simulink model "clase3"  (R2022b)
settings: Solver=VariableStepAuto  StartTime=0.0  StopTime=10  MaxStep=0.01  RelTol=1e-3
values from neighbouring files (symbols this model uses):
  g = 9.81    [class3.m]
  l1 = 0.3    [class3.m]
  l2 = 0.25    [class3.m]
  m1 = 0.2    [class3.m]
  m2 = 0.1    [class3.m]
settings Model: Creator=nemesis  LastModifiedBy=nemesis

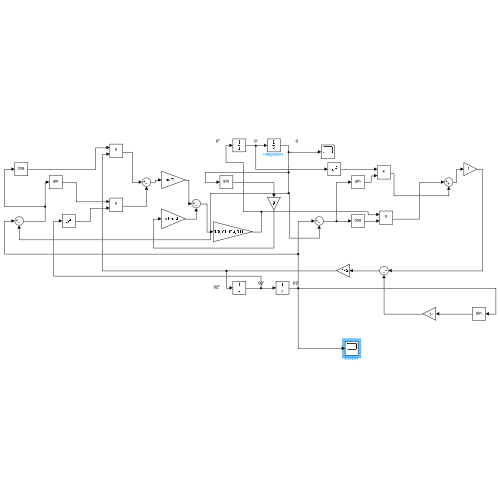
[thumbnail: Simulink's stored preview of the top-level diagram]
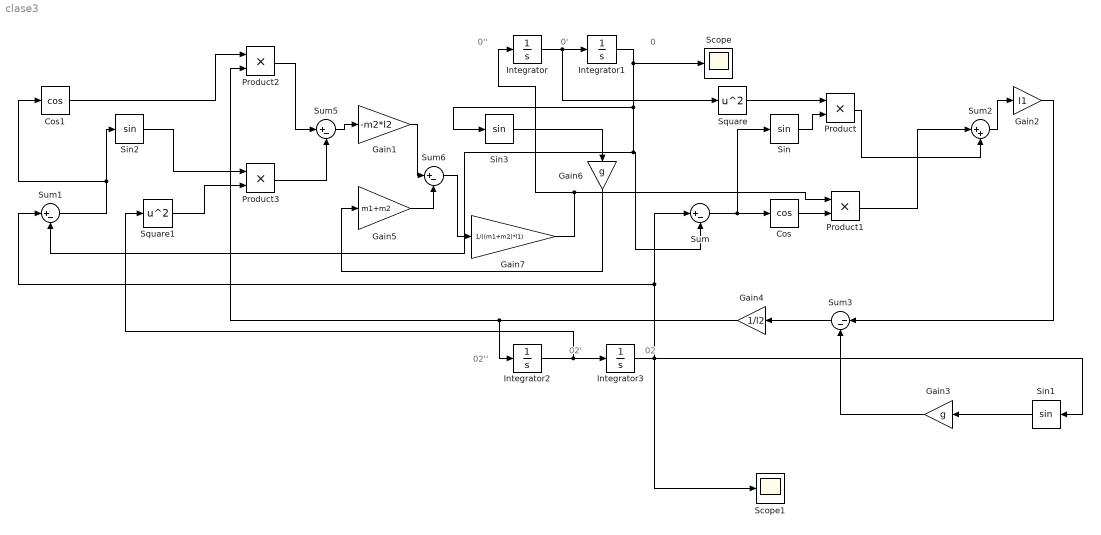
== system clase3 ==
  note: 02''
  note: 0''
  note: 0'
  note: 0
  note: 02'
  note: 02
  Cos : Trigonometry  Operator=cos
  Cos1 : Trigonometry  Operator=cos
  Gain1 : Gain  Gain=-m2*l2
  Gain2 : Gain  Gain=l1
  Gain3 : Gain  Gain=g
  Gain4 : Gain  Gain=1/l2
  Gain5 : Gain  Gain=m1+m2
  Gain6 : Gain  Gain=g
  Gain7 : Gain  Gain=1/((m1+m2)*l1)
  Integrator : Integrator
  Integrator1 : Integrator
  Integrator2 : Integrator
  Integrator3 : Integrator  InitialCondition=(35*pi)/180
  Product{,1..3} (4 alike) : Product
  Scope : Scope
  Scope1 : Scope
  Sin{,1..3} (4 alike) : Trigonometry
  Square : Math  Operator=square
  Square1 : Math  Operator=square
  Sum{,1,5..6} (4 alike) : Sum  Inputs=|+-
  Sum2 : Sum  Inputs=|++
  Sum3 : Sum  Inputs=|--
  wires:
  Integrator/1 -> Square/1, Integrator1/1
  Sum3/1 -> Gain4/1
  Integrator2/1 -> Square1/1, Integrator3/1
  Integrator1/1 -> Scope/1, Sum/2, Sum1/2, Sin3/1
  Integrator3/1 -> Scope1/1, Sum/1, Sum1/1, Sin1/1
  Sum/1 -> Sin/1, Cos/1
  Square/1 -> Product/1
  Sin/1 -> Product/2
  Cos/1 -> Product1/2
  Product/1 -> Sum2/2
  Product1/1 -> Sum2/1
  Sum2/1 -> Gain2/1
  Sin1/1 -> Gain3/1
  Gain2/1 -> Sum3/1
  Gain3/1 -> Sum3/2
  Gain4/1 -> Product2/2, Integrator2/1
  Cos1/1 -> Product2/1
  Sum1/1 -> Cos1/1, Sin2/1
  Sin2/1 -> Product3/1
  Square1/1 -> Product3/2
  Product2/1 -> Sum5/1
  Product3/1 -> Sum5/2
  Sum5/1 -> Gain1/1
  Sin3/1 -> Gain6/1
  Gain6/1 -> Gain5/1
  Gain5/1 -> Sum6/2
  Gain1/1 -> Sum6/1
  Sum6/1 -> Gain7/1
  Gain7/1 -> Integrator/1, Product1/1
